simulink model "interactiveRobotLIPM"  (R2023b)
settings: Solver=ode15s  StartTime=0.0  StopTime=inf  EnableMultiTasking=on
PreLoadFcn:
  | robotParameters
  | load('defaultsimulationinputs.mat')
undefined symbols (not defined in the file): torso_width
libraries: walkingRobotUtils x4, simulink x1
settings Model: Creator=bkim  LastModifiedBy=samradny
settings SolverCC: AlgebraicLoopSolver=TrustRegion
settings DataIOCC: ReturnWorkspaceOutputs=off  OutputSaveName=simout  OutputTimes=0:0.01:10
settings OptimizationCC: LifeSpan=inf
settings DebuggingCC: UnconnectedInputMsg=warning  UnconnectedOutputMsg=warning  UnconnectedLineMsg=warning  AllowSymbolicDim=off  PregeneratedLibrarySubsystemCodeDiagnostic=none  SFUnexpectedBacktrackingDiag=warning  SFNoUnconditionalDefaultTransitionDiag=warning  SFExecutionAtInitializationDiag=none  UnitsInconsistencyMsg=none  ArithmeticOperatorsInVariantConditions=warning
settings ModelReferenceCC: EnableRefExpFcnMdlSchedulingChecks=on
settings SFSimCC: SimUseLocalCustomCode=off  CustomCodeUndefinedFunction=UseInterfaceOnly
settings RTWCC: RTWUseLocalCustomCode=off
settings CodeAppCC: StateflowObjectComments=on
settings GRTTargetCC: TargetLangStandard=C89/C90 (ANSI)
settings ConfigComp: CovMetricSettings=dw  CovSaveCumulativeToWorkspaceVar=on  CovSaveSingleToWorkspaceVar=on  CovExternalEMLEnable=off  CovSFcnEnable=off
settings SimscapeCC: SimscapeNormalizeSystem=off  SimscapeLogOpenViewer=on  SimscapeLogLimitData=off  SimscapeLogDataHistory=10000
settings ConfigurationSet: Description=SimMechanics 2G
settings DiagnosticsConfigSet: SimMechanicsRigidlyBoundBlock=none
settings ExplorerConfigSet: InternalSimMechanicsExplorerSettings="<ExplorerConfiguration><canonicalview>default</canonicalview><AnimationSetting><BasePlaybackSpeed>1.0</BasePlaybackSpeed><PlaybackSpeedFactor>1.0</PlaybackSpeedFactor></AnimationSetting><TilePanel><TileInfo><Tiles Columns=\"1\" Count=\"1\" Rows=\"1\"><Column Weight=\"1\"/><Row Weight=\"1\"/><Tile Height=\"1\" Width=\"1\" X=\"0\" Y=\"0\"/></Tiles></TileInfo><SceneInfo><SceneViewer><BGColor><R>0.60000002384185791</R><G>0.60000002384185791</G><B>0.60000002384185791</B></BGColor><Camera><DoPerspective>off</DoPerspective><Position><X>-9.25260698060568743</X><Y>23.845286333652421</Y><Z>5.02226343405862519</Z></Position><Center><X>-0.867112304450580074</X><Y>0.122914316828580963</Y><Z>0.414972701616938722</Z></Center><Up><X>0.114101071913408486</X><Y>-0.150392103718327563</Y><Z>0.982019938966306238</Z></Up><ViewLimDist>1</ViewLimDist><YLim>2.27758996587981333</YLim><XLim>2.91728344395099537</XLim></Camera></SceneViewer></SceneInfo></TilePanel><MechEditorPanel><Cameras/><GfxPanelCameraMap/><VideoCreator><PlaybackSpeedRatio>1.0</PlaybackSpeedRatio><FrameRate>30</FrameRate><VideoFormat>Motion JPEG AVI</VideoFormat><FrameSize>auto</FrameSize></VideoCreator></MechEditorPanel></ExplorerConfiguration>"

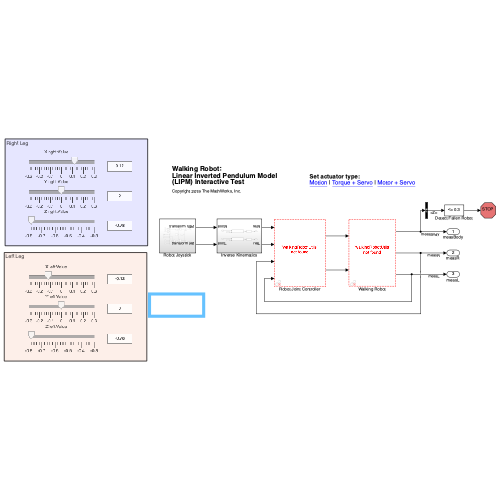
[thumbnail: Simulink's stored preview of the top-level diagram]
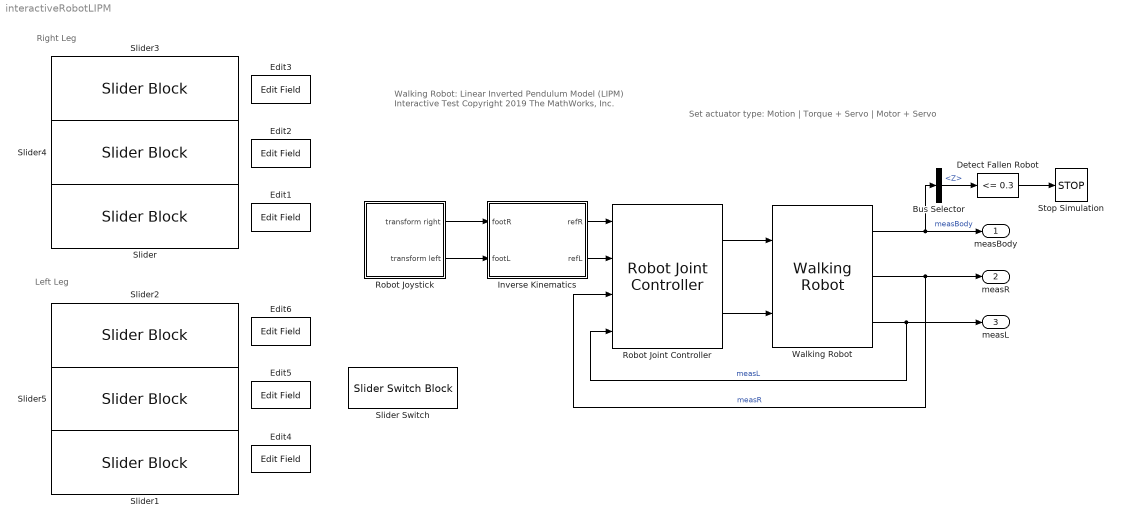
== system interactiveRobotLIPM ==
  note: Left Leg
  note: Right Leg
  note: Walking Robot:
      | Linear Inverted Pendulum Model (LIPM) Interactive Test
      |
      | Copyright 2019 The MathWorks, Inc.
  note: Set actuator type:
      | Motion | Torque + Servo | Motor + Servo
  Bus Selector : BusSelector  OutputSignals=Z
  Detect Fallen Robot : simulink/Logic and Bit Operations/Compare To Constant  relop=<=  const=0.3  OutDataTypeStr=boolean
  Edit{1..6} (6 alike) : EditField  LabelPosition=Hide  ShowInitialText=on  Alignment=Center
  Inverse Kinematics : Subsystem
  Robot Joint Controller : walkingRobotUtils/Robot Joint Controller  SystemSampleTime=-1  Latency=0  AutoFrameSizeCalculation=off
  Robot Joystick : Subsystem
  Slider : SliderBlock  ScaleMin=-0.8  ScaleMax=-0.3
  Slider Switch : SliderSwitchBlock
      settings: Values={{'Off', 'On'}, [0 1]}
  Slider1 : SliderBlock  ScaleMin=-0.8  ScaleMax=-0.3
  Slider{2..5} (4 alike) : SliderBlock  ScaleMin=-0.3  ScaleMax=0.3
  Stop Simulation : Stop
  Walking Robot : walkingRobotUtils/Walking Robot  SystemSampleTime=-1  Latency=0  AutoFrameSizeCalculation=off
  measBody : Outport  VectorParamsAs1DForOutWhenUnconnected=off
  measR : Outport  Port=2  VectorParamsAs1DForOutWhenUnconnected=off
  measL : Outport  Port=3  VectorParamsAs1DForOutWhenUnconnected=off
  wires:
  Robot Joint Controller/1 -> Walking Robot/1
  Walking Robot/3 -> Robot Joint Controller/4, measL/1  "measL"
  Walking Robot/2 -> Robot Joint Controller/3, measR/1  "measR"
  Inverse Kinematics/1(refR) -> Robot Joint Controller/1
  Inverse Kinematics/2(refL) -> Robot Joint Controller/2
  Detect Fallen Robot/1 -> Stop Simulation/1
  Walking Robot/1 -> Bus Selector/1, measBody/1  "measBody"
  Robot Joystick/2(transform left) -> Inverse Kinematics/2(footL)
  Robot Joint Controller/2 -> Walking Robot/2
  Robot Joystick/1(transform right) -> Inverse Kinematics/1(footR)
  Bus Selector/1 -> Detect Fallen Robot/1  "<Z>"

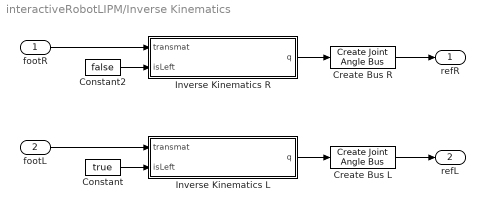
== system interactiveRobotLIPM/Inverse Kinematics ==
  footR : Inport
  footL : Inport  Port=2
  Constant : Constant  Value=true
  Constant2 : Constant  Value=false
  Create Bus L : walkingRobotUtils/Create Joint Angle Bus  SystemSampleTime=-1  Latency=0  AutoFrameSizeCalculation=off
  Create Bus R : walkingRobotUtils/Create Joint Angle Bus  SystemSampleTime=-1  Latency=0  AutoFrameSizeCalculation=off
  Inverse Kinematics L : MATLAB Function  TreatAsAtomicUnit=on
  Inverse Kinematics R : MATLAB Function  TreatAsAtomicUnit=on
  refR : Outport
  refL : Outport  Port=2
  wires:
  footR/1 -> Inverse Kinematics R/1(transmat)
  Inverse Kinematics L/1(q) -> Create Bus L/1
  Constant2/1 -> Inverse Kinematics R/2(isLeft)
  Create Bus R/1 -> refR/1
  Create Bus L/1 -> refL/1
  Constant/1 -> Inverse Kinematics L/2(isLeft)
  Inverse Kinematics R/1(q) -> Create Bus R/1
  footL/1 -> Inverse Kinematics L/1(transmat)

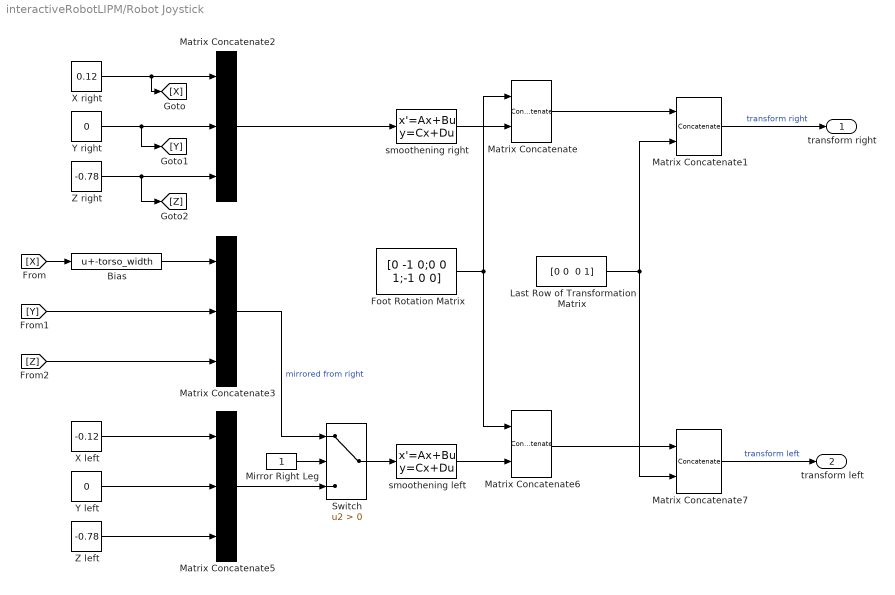
== system interactiveRobotLIPM/Robot Joystick ==
  Bias : Bias  Bias=-torso_width  SaturateOnIntegerOverflow=off
  Foot Rotation Matrix : Constant  Value=[0 -1 0;0 0 1;-1 0 0]
  Last Row of Transformation Matrix : Constant  Value="[0 0  0 1]"  VectorParams1D=off
  Matrix Concatenate : Concatenate  Mode=Multidimensional array  ConcatenateDimension=2
  Matrix Concatenate1 : Concatenate  Mode=Multidimensional array
  Matrix Concatenate2 : Concatenate  NumInputs=3  Mode=Multidimensional array
  Matrix Concatenate3 : Concatenate  NumInputs=3  Mode=Multidimensional array
  Matrix Concatenate5 : Concatenate  NumInputs=3  Mode=Multidimensional array
  Matrix Concatenate6 : Concatenate  Mode=Multidimensional array  ConcatenateDimension=2
  Matrix Concatenate7 : Concatenate  Mode=Multidimensional array
  Mirror Right Leg : Constant  InitFcn=set_param(gcb, 'Value', '1');
  Switch : Switch  Criteria=u2 > Threshold  SaturateOnIntegerOverflow=off  InputSameDT=off
  X left : Constant  InitFcn=set_param(gcb, 'Value', '-0.12');  Value=-0.12
  X right : Constant  InitFcn=set_param(gcb, 'Value', '0.12');  Value=0.12
  Y left : Constant  InitFcn=set_param(gcb, 'Value', '0');  Value=0
  Y right : Constant  InitFcn=set_param(gcb, 'Value', '0');  Value=0
  Z left : Constant  InitFcn=set_param(gcb, 'Value', '-0.78');  Value=-0.78
  Z right : Constant  InitFcn=set_param(gcb, 'Value', '-0.78');  Value=-0.78
  smoothening left : StateSpace  A=-1*eye(3)  B=eye(3)  C=eye(3)  D=zeros(3)  InitialCondition=[-0.12 0 -0.78]
  smoothening right : StateSpace  A=-1*eye(3)  B=eye(3)  C=eye(3)  D=zeros(3)  InitialCondition=[0.12 0 -0.78]
  transform right : Outport
  transform left : Outport  Port=2
  wires:
  Z left/1 -> Matrix Concatenate5/3
  [X] -> Bias/1
  Last Row of Transformation Matrix/1 -> Matrix Concatenate1/2, Matrix Concatenate7/2
  Y right/1 -> Matrix Concatenate2/2, [Y]
  Matrix Concatenate3/1 -> Switch/1  "mirrored from right"
  Foot Rotation Matrix/1 -> Matrix Concatenate/1, Matrix Concatenate6/1
  Bias/1 -> Matrix Concatenate3/1
  smoothening left/1 -> Matrix Concatenate6/2
  Matrix Concatenate1/1 -> transform right/1  "transform right"
  Matrix Concatenate/1 -> Matrix Concatenate1/1
  Z right/1 -> Matrix Concatenate2/3, [Z]
  Matrix Concatenate7/1 -> transform left/1  "transform left"
  X right/1 -> [X], Matrix Concatenate2/1
  Matrix Concatenate5/1 -> Switch/3
  [Z] -> Matrix Concatenate3/3
  Matrix Concatenate6/1 -> Matrix Concatenate7/1
  X left/1 -> Matrix Concatenate5/1
  [Y] -> Matrix Concatenate3/2
  Y left/1 -> Matrix Concatenate5/2
  Matrix Concatenate2/1 -> smoothening right/1
  smoothening right/1 -> Matrix Concatenate/2
  Switch/1 -> smoothening left/1
  Mirror Right Leg/1 -> Switch/2

== matlab function interactiveRobotLIPM/Inverse Kinematics/Inverse Kinematics R ==
  data: transmat input; q output; isLeft input
function q = inverseKinematics(transmat, isLeft)
q = invKinBody2Foot(transmat, isLeft);

== matlab function interactiveRobotLIPM/Inverse Kinematics/Inverse Kinematics L ==
  data: transmat input; q output; isLeft input
function q = inverseKinematics(transmat, isLeft)
q = invKinBody2Foot(transmat, isLeft);
